simulink model "car_model"  (R2017a)
settings: Solver=ode8  StartTime=0.0  StopTime=tf  FixedStep=1e-3  RelTol=1e-3  AbsTol=1e-6
values from neighbouring files (symbols this model uses):
  L = sys.descrip.syms(end-2)    [load_consts.m]    (also in run_sim.m = sys.descrip.model_params(end-2))
  MAX_DELTA = deg2rad(MAX_DELTA)    [run_sim.m]
  w = sys.descrip.syms(end-3)    [load_consts.m]    (also in run_sim.m = sys.descrip.model_params(end-3))
  x0 = double(subs([qs0; ps0], symbs, vals))    [run_sim.m]
undefined symbols (not defined in the file or in its folder): sys
settings Model: Creator=brunolnetto  LastModifiedBy=brunolnetto
settings DataIOCC: SaveState=on  StateSaveName=xoutNew  OutputSaveName=youtNew

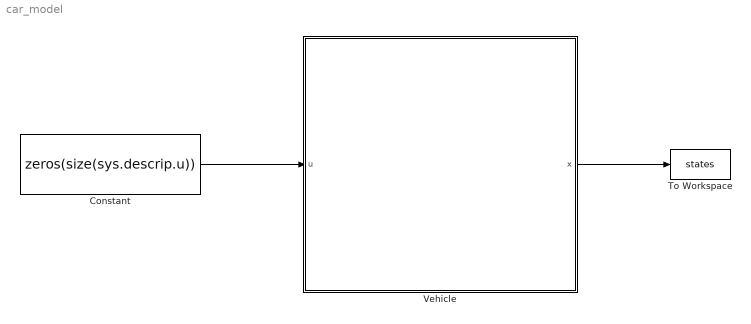
== system car_model ==
  Constant : Constant  Value=zeros(size(sys.descrip.u))
  To Workspace : ToWorkspace  VariableName=states  SaveFormat=Structure With Time  SampleTime=-1
  Vehicle : Subsystem
      mask Display: image('/home/brunolnetto/Pictures/auto_model.png');
  wires:
  Constant/1 -> Vehicle/1(u)
  Vehicle/1(x) -> To Workspace/1

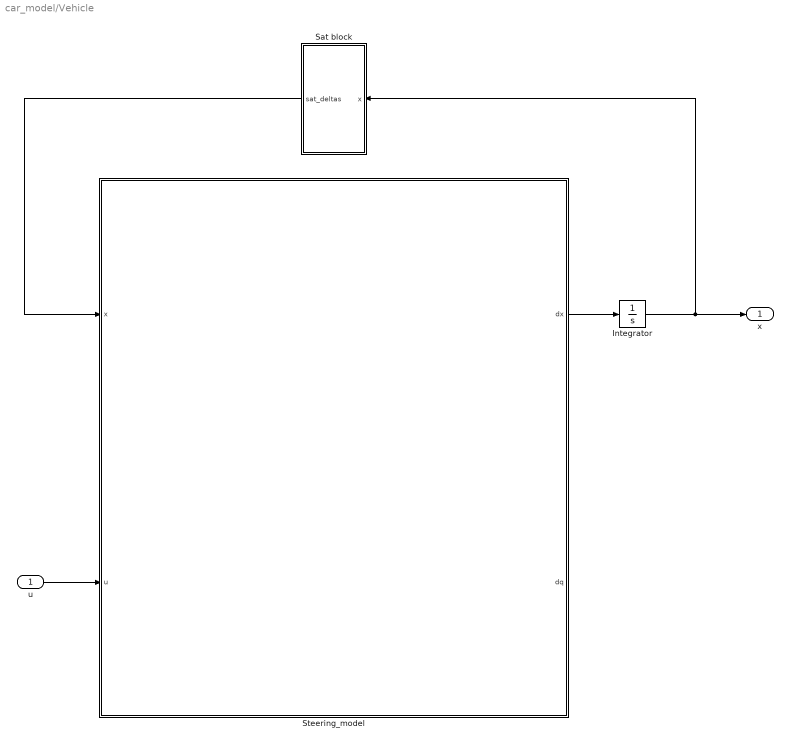
== system car_model/Vehicle ==
  u : Inport
  Integrator : Integrator  InitialCondition=x0
  Sat block : Subsystem
  Steering_model : Subsystem
      mask Display: image('/home/brunolnetto/Pictures/steer_schema.png');
  x : Outport
  wires:
  Steering_model/1(dx) -> Integrator/1
  u/1 -> Steering_model/2(u)
  Integrator/1 -> Sat block/1(x), x/1
  Sat block/1(sat_deltas) -> Steering_model/1(x)

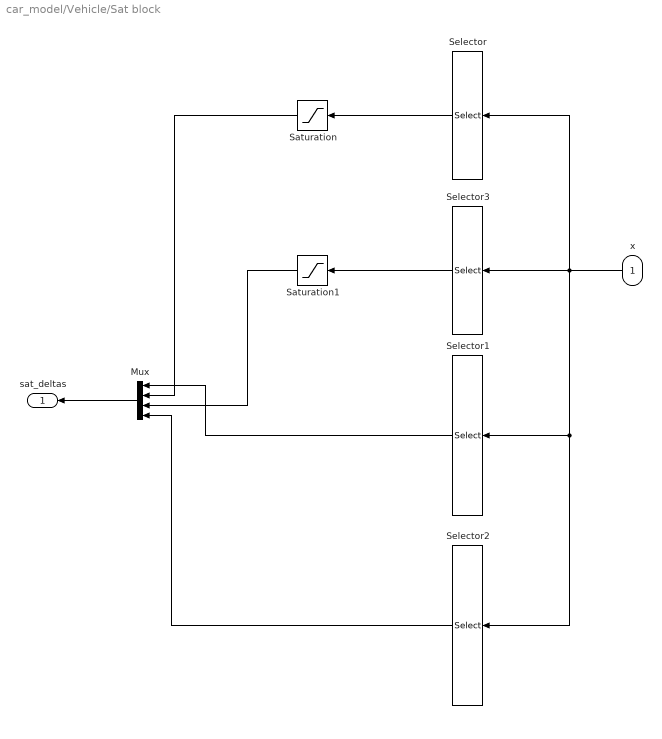
== system car_model/Vehicle/Sat block ==
  x : Inport
  Mux : Mux
  Saturation : Saturate  UpperLimit=MAX_DELTA  LowerLimit=atan(tan(-MAX_DELTA)/(1 - (w/L)*tan(-MAX_DELTA)))  LinearizeAsGain=off
  Saturation1 : Saturate  UpperLimit=atan(tan(MAX_DELTA)/(1 + (w/L)*tan(MAX_DELTA)))  LowerLimit=-MAX_DELTA  LinearizeAsGain=off
  Selector : Selector  InputPortWidth=length(x0)  IndexOptions=Index vector (dialog)  Indices=4  OutputSizes=1
  Selector1 : Selector  InputPortWidth=length(x0)  IndexOptions=Index vector (dialog)  Indices=[1 2. 3]  OutputSizes=1
  Selector2 : Selector  InputPortWidth=length(x0)  IndexOptions=Index vector (dialog)  Indices=6:length(x0)  OutputSizes=1
  Selector3 : Selector  InputPortWidth=length(x0)  IndexOptions=Index vector (dialog)  Indices=5  OutputSizes=1
  sat_deltas : Outport
  wires:
  Mux/1 -> sat_deltas/1
  x/1 -> Selector2/1, Selector1/1, Selector3/1, Selector/1
  Selector2/1 -> Mux/4
  Selector1/1 -> Mux/1
  Selector/1 -> Saturation/1
  Saturation/1 -> Mux/2
  Saturation1/1 -> Mux/3
  Selector3/1 -> Saturation1/1

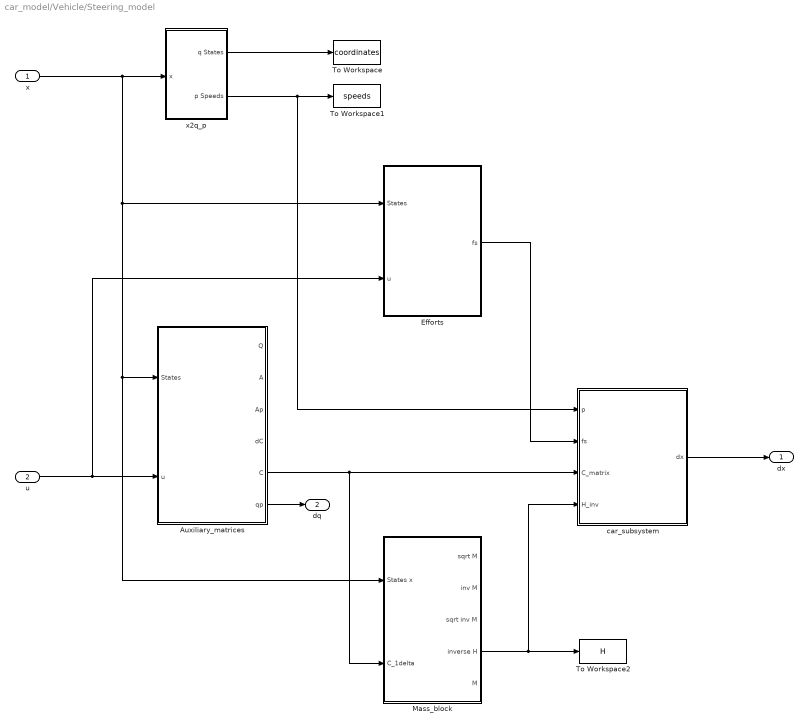
== system car_model/Vehicle/Steering_model ==
  x : Inport
  u : Inport  Port=2
  Auxiliary_matrices : Subsystem
  Efforts : Subsystem
  Mass_block : Subsystem
  To Workspace : ToWorkspace  VariableName=coordinates  SaveFormat=Structure With Time  SampleTime=-1
  To Workspace1 : ToWorkspace  VariableName=speeds  SaveFormat=Structure With Time  SampleTime=-1
  To Workspace2 : ToWorkspace  VariableName=H  SaveFormat=Structure With Time  SampleTime=-1
  car_subsystem : Subsystem
  x2q_p : Subsystem
  dx : Outport
  dq : Outport  Port=2
  wires:
  Auxiliary_matrices/5(C) -> Mass_block/2("C_1delta  "), car_subsystem/3(C_matrix)
  u/1 -> Efforts/2(u), Auxiliary_matrices/2(u)
  Mass_block/4(inverse H) -> To Workspace2/1, car_subsystem/4(H_inv)
  car_subsystem/1(dx) -> dx/1
  Efforts/1(fs) -> car_subsystem/2(fs)
  x2q_p/1(q States) -> To Workspace/1
  x2q_p/2(p Speeds) -> To Workspace1/1, car_subsystem/1(p)
  x/1 -> x2q_p/1(x), Mass_block/1(States x), Auxiliary_matrices/1(States), Efforts/1(States)
  Auxiliary_matrices/6(qp) -> dq/1

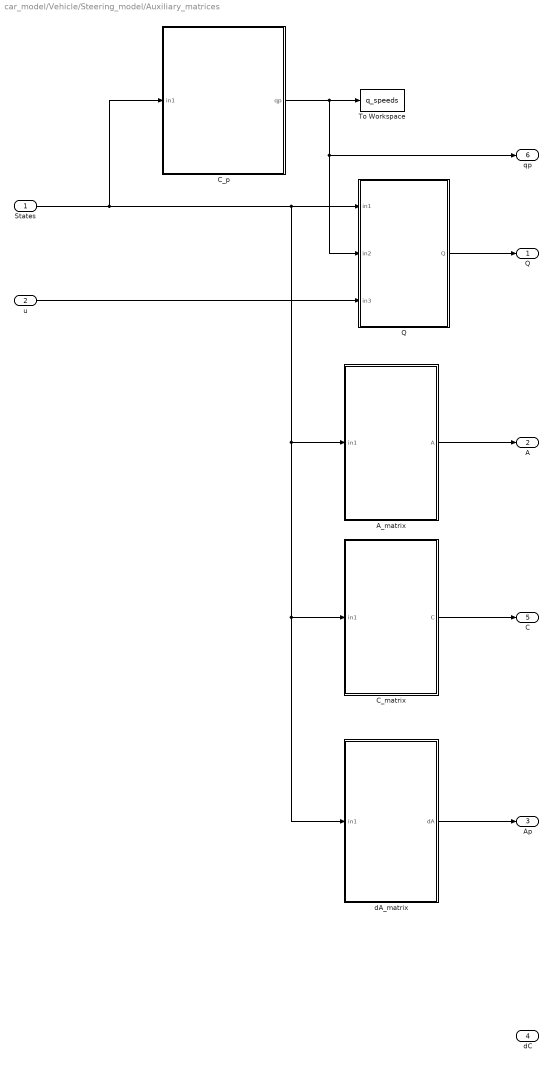
== system car_model/Vehicle/Steering_model/Auxiliary_matrices ==
  States : Inport
  u : Inport  Port=2
  A_matrix : MATLAB Function  TreatAsAtomicUnit=on
  C_matrix : MATLAB Function  TreatAsAtomicUnit=on
  C_p : MATLAB Function  TreatAsAtomicUnit=on
  Q : MATLAB Function  TreatAsAtomicUnit=on
  To Workspace : ToWorkspace  VariableName=q_speeds  SaveFormat=Structure With Time  SampleTime=-1
  dA_matrix : MATLAB Function  TreatAsAtomicUnit=on
  "Q " : Outport
  A : Outport  Port=2
  Ap : Outport  Port=3
  dC : Outport  Port=4
  C : Outport  Port=5
  qp : Outport  Port=6
  wires:
  C_matrix/1(C) -> C/1
  Q/1(Q) -> "Q "/1
  A_matrix/1(A) -> A/1
  dA_matrix/1(dA) -> Ap/1
  u/1 -> Q/3(in3)
  States/1 -> C_p/1(in1), dA_matrix/1(in1), C_matrix/1(in1), A_matrix/1(in1), Q/1(in1)
  C_p/1(qp) -> To Workspace/1, qp/1, Q/2(in2)

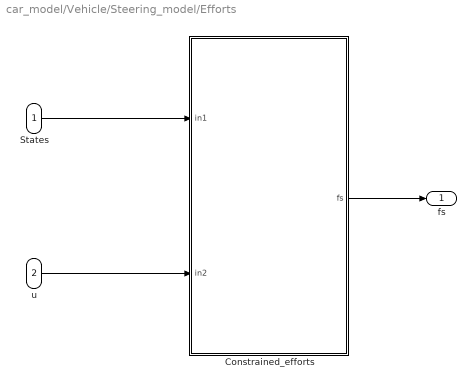
== system car_model/Vehicle/Steering_model/Efforts ==
  States : Inport
  u : Inport  Port=2
  Constrained_efforts : MATLAB Function  TreatAsAtomicUnit=on
  fs : Outport
  wires:
  States/1 -> Constrained_efforts/1(in1)
  u/1 -> Constrained_efforts/2(in2)
  Constrained_efforts/1(fs) -> fs/1

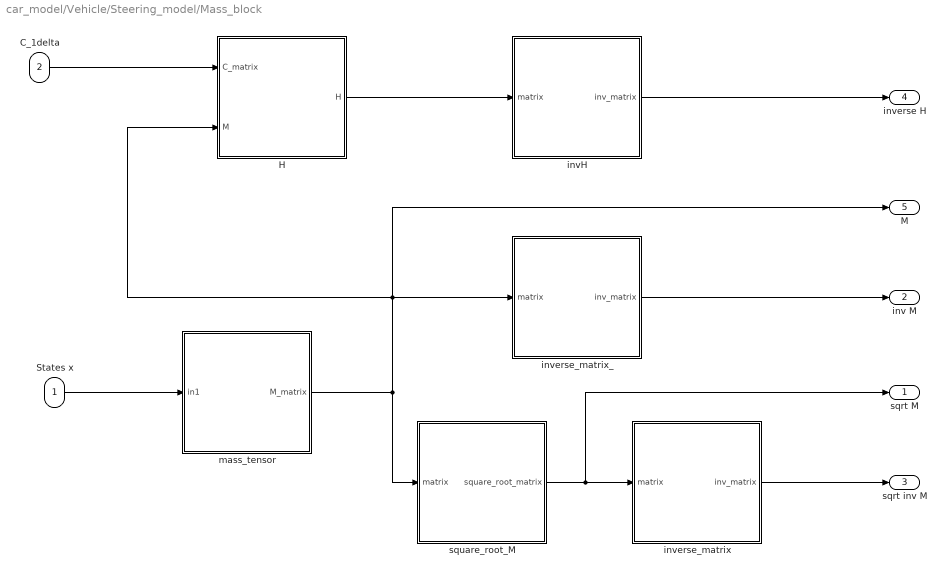
== system car_model/Vehicle/Steering_model/Mass_block ==
  States x : Inport
  "C_1delta  " : Inport  Port=2
  H : MATLAB Function  TreatAsAtomicUnit=on
  invH : MATLAB Function  TreatAsAtomicUnit=on
  inverse_matrix : MATLAB Function  TreatAsAtomicUnit=on
  inverse_matrix_ : MATLAB Function  TreatAsAtomicUnit=on
  mass_tensor : MATLAB Function  TreatAsAtomicUnit=on
  square_root_M : MATLAB Function  TreatAsAtomicUnit=on
  sqrt M : Outport
  inv M : Outport  Port=2
  sqrt inv M : Outport  Port=3
  inverse H : Outport  Port=4
  M : Outport  Port=5
  wires:
  States x/1 -> mass_tensor/1(in1)
  "C_1delta  "/1 -> H/1(C_matrix)
  inverse_matrix_/1(inv_matrix) -> inv M/1
  H/1(H) -> invH/1(matrix)
  invH/1(inv_matrix) -> inverse H/1
  inverse_matrix/1(inv_matrix) -> sqrt inv M/1
  mass_tensor/1(M_matrix) -> M/1, inverse_matrix_/1(matrix), H/2(M), square_root_M/1(matrix)
  square_root_M/1(square_root_matrix) -> sqrt M/1, inverse_matrix/1(matrix)

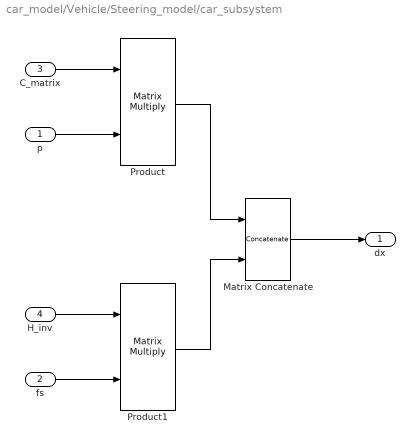
== system car_model/Vehicle/Steering_model/car_subsystem ==
  p : Inport
  fs : Inport  Port=2
  C_matrix : Inport  Port=3
  H_inv : Inport  Port=4
  Matrix Concatenate : Concatenate  ConcatenateDimension=2
  Product : Product  Multiplication=Matrix(*)
  Product1 : Product  Multiplication=Matrix(*)
  dx : Outport
  wires:
  Product/1 -> Matrix Concatenate/1
  p/1 -> Product/2
  C_matrix/1 -> Product/1
  Product1/1 -> Matrix Concatenate/2
  H_inv/1 -> Product1/1
  fs/1 -> Product1/2
  Matrix Concatenate/1 -> dx/1

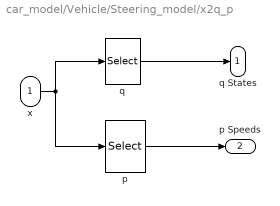
== system car_model/Vehicle/Steering_model/x2q_p ==
  x : Inport
  p : Selector  InputPortWidth=length(sys.kin.q) + length(sys.kin.p{end})  IndexOptions=Index vector (dialog)  Indices=length(sys.kin.q)+1:length(sys.kin.q) + length(sys.kin.p{end})  OutputSizes=1
  q : Selector  InputPortWidth=length(sys.kin.q) + length(sys.kin.p{end})  IndexOptions=Index vector (dialog)  Indices=1:length(sys.kin.q)  OutputSizes=1
  q States : Outport
  p Speeds : Outport  Port=2
  wires:
  x/1 -> p/1, q/1
  q/1 -> q States/1
  p/1 -> p Speeds/1

== matlab function car_model/Vehicle/Steering_model/Auxiliary_matrices/A_matrix ==
  data: in1 input; A output
function A = ConstraintMatrix(in1)

%    This function was generated by the Symbolic Math Toolbox version 7.2.

%    01-Dec-2020 16:45:13



delta_i = in1(4,:);

theta = in1(3,:);

t2 = tan(delta_i);

t3 = t2.*(3.0./2.0);

t4 = t3+9.0./2.0;

t5 = t2.^2;

t6 = t2.*(1.0./6.0);

t7 = t6+1.0;

t8 = 1.0./t7;

t9 = t2.*t8;

t10 = atan(t9);

t11 = t10.*2.0;

t12 = t11+theta;

t13 = 1.0./t4.^2;

t14 = t5.*t13.*(8.1e1./4.0);

t15 = t14+1.0;

t16 = cos(delta_i);

t17 = t16.*(9.0./2.0);

t18 = sin(delta_i);

t19 = t18.*(3.0./2.0);

t20 = t17+t19;

t21 = delta_i+theta;

t22 = sin(t21);

t23 = cos(t21);

A = reshape([0.0,cos(t12).*(-9.0./2.0)-cos(theta).*(9.0./2.0),0.0,0.0,0.0,t23,-t22,0.0,sin(t12).*(-9.0./2.0)-sin(theta).*(9.0./2.0),0.0,0.0,0.0,t22,t23,0.0,sin(t11).*(-8.1e1./8.0),0.0,0.0,0.0,-t17-t18.*(3.0./4.0),t16.*(-3.0./4.0)+t18.*(9.0./2.0),((t2.*(2.7e1./4.0))./t4-9.0./2.0).*(t5+1.0).*(-2.0./9.0),0.0,0.0,0.0,0.0,0.0,0.0,t4.*t15.*(-2.0./9.0),0.0,0.0,0.0,0.0,0.0,0.0,0.0,0.0,t20,0.0,t20,-3.442462000000001e-1,0.0,0.0,0.0,1.0./sqrt(t15).*(-9.0./2.0),0.0,0.0,0.0,0.0,0.0,0.0,0.0,-9.0./2.0,-9.0./2.0,0.0,0.0,0.0,t2.*5.163693000000001e-1+3.098215800000001,0.0,t4,0.0,0.0,0.0],[7,9]);

end

== matlab function car_model/Vehicle/Steering_model/Mass_block/mass_tensor ==
  data: in1 input; M_matrix output
function M_matrix = Mass_matrix(in1)

%    This function was generated by the Symbolic Math Toolbox version 7.2.

%    01-Dec-2020 16:45:20



phi_i = in1(6,:);

phi_l = in1(9,:);

phi_o = in1(7,:);

phi_r = in1(8,:);

theta = in1(3,:);

t2 = cos(theta);

t3 = sin(theta);

t4 = cos(phi_i);

t5 = cos(phi_l);

t6 = cos(phi_o);

t7 = cos(phi_r);

t8 = t4.^2;

t9 = sin(phi_i);

t10 = t6.^2;

t11 = sin(phi_o);

t12 = t8.*4.147690617505401e-1;

t13 = t9.^2;

t14 = t13.*2.073845308752701e-1;

t15 = t12+t14;

t16 = t10.*4.147690617505401e-1;

t17 = t11.^2;

t18 = t17.*2.073845308752701e-1;

t19 = t16+t18;

M_matrix = reshape([1.885e3,0.0,t2.*(-4.24125e3),0.0,0.0,0.0,0.0,0.0,0.0,0.0,1.885e3,t3.*(-4.24125e3),0.0,0.0,0.0,0.0,0.0,0.0,t2.*(-4.24125e3),t3.*(-4.24125e3),t8.*2.073845308752701e-1+t10.*2.073845308752701e-1+t5.^2.*2.073845308752701e-1+t7.^2.*2.073845308752701e-1+1.31830170381235e4,t15,t19,0.0,0.0,0.0,0.0,0.0,0.0,t15,t15,0.0,0.0,0.0,0.0,0.0,0.0,0.0,t19,0.0,t19,0.0,0.0,0.0,0.0,0.0,0.0,0.0,0.0,0.0,2.073845308752701e-1,0.0,0.0,0.0,0.0,0.0,0.0,0.0,0.0,0.0,2.073845308752701e-1,0.0,0.0,0.0,0.0,0.0,0.0,0.0,0.0,0.0,2.073845308752701e-1,0.0,0.0,0.0,0.0,0.0,0.0,0.0,0.0,0.0,2.073845308752701e-1],[9,9]);

end

== matlab function car_model/Vehicle/Steering_model/Auxiliary_matrices/C_matrix ==
  data: in1 input; C output
function C = KinematicMatrix(in1)

%    This function was generated by the Symbolic Math Toolbox version 7.2.

%    01-Dec-2020 16:45:15



delta_i = in1(4,:);

theta = in1(3,:);

t2 = sin(delta_i);

t3 = tan(delta_i);

t4 = delta_i+theta;

t5 = cos(delta_i);

t6 = sin(theta);

t7 = t3.^2;

t8 = t3.*(1.0./6.0);

t9 = t8+1.0;

t10 = 1.0./t9.^2;

t11 = t7.*t10;

t12 = t11+1.0;

t13 = 1.0./t12;

t14 = sin(t4);

t15 = cos(t4);

t16 = cos(theta);

t17 = t16.^2;

t18 = 1.0./t9;

t19 = t15.^2;

t20 = t14.^2;

t21 = t6.^2;

t22 = t5.^2;

t23 = t2.^2;

t24 = t5.*(9.0./2.0);

t25 = t2.*(3.0./2.0);

t26 = t24+t25;

t27 = 1.0./t26;

t28 = t5.*t6.*t13.*t14.*(8.1e1./2.0);

t29 = t2.*t13.*t14.*t16.*(8.1e1./2.0);

t30 = t2.*t6.*t13.*t14.*(2.7e1./4.0);

t31 = t5.*t13.*t15.*t16.*(8.1e1./2.0);

t32 = t5.*t6.*t13.*t15.*(2.7e1./4.0);

t33 = t2.*t13.*t15.*t16.*(2.7e1./4.0);

t34 = t3.*t13.*t17.*t18.*t19.*(8.1e1./4.0);

t35 = t3.*t13.*t17.*t18.*t20.*(8.1e1./4.0);

t36 = t3.*t13.*t18.*t19.*t21.*(8.1e1./4.0);

t37 = t3.*t13.*t18.*t20.*t21.*(8.1e1./4.0);

t38 = t3.*t5.*t13.*t15.*t16.*t18.*(2.7e1./4.0);

t39 = t3.*t5.*t13.*t14.*t16.*t18.*(8.1e1./2.0);

t40 = t3.*t5.*t6.*t13.*t14.*t18.*(2.7e1./4.0);

t41 = t2.*t3.*t13.*t14.*t16.*t18.*(2.7e1./4.0);

t44 = t2.*t6.*t13.*t15.*(8.1e1./2.0);

t45 = t5.*t13.*t14.*t16.*(2.7e1./4.0);

t46 = t3.*t5.*t6.*t13.*t15.*t18.*(8.1e1./2.0);

t47 = t2.*t3.*t13.*t15.*t16.*t18.*(8.1e1./2.0);

t48 = t2.*t3.*t6.*t13.*t15.*t18.*(2.7e1./4.0);

t49 = t2.*t3.*t6.*t13.*t14.*t18.*(8.1e1./2.0);

t42 = t28+t29+t30+t31+t32+t33+t34+t35+t36+t37+t38+t39+t40+t41-t44-t45-t46-t47-t48-t49;

t43 = 1.0./t42;

t50 = t3.*(3.0./2.0);

t51 = t50+9.0./2.0;

t52 = 1.0./t51;

t53 = 1.0./t51.^2;

C = reshape([0.0,0.0,0.0,(t50+t7.*t53.*(7.29e2./8.0)+t3.*t7.*t53.*(2.43e2./8.0)+9.0./2.0)./(t7.*(9.0./2.0)-t3.*t52.*(2.7e1./4.0)-t3.*t7.*t52.*(2.7e1./4.0)+9.0./2.0),1.0,0.0,0.0,0.0,0.0,t27.*t43.*(t14.*t22.*(-2.091295665e1)+t14.*t23.*4.182591330000001e1+t15.*t22.*1.254777399e2+t15.*t23.*6.970985550000001+t2.*t5.*t14.*1.1850675435e2-t2.*t6.*t13.*1.254777399e2+t2.*t5.*t15.*6.273886995000001e1+t5.*t6.*t13.*2.091295665e1-t3.*t14.*t22.*3.485492775000001+t3.*t14.*t23.*6.970985550000001+t3.*t15.*t22.*2.091295665e1+t3.*t15.*t23.*1.161830925+t2.*t3.*t5.*t14.*1.9751125725e1-t2.*t3.*t6.*t13.*4.182591330000001e1+t2.*t3.*t5.*t15.*1.0456478325e1+t3.*t5.*t6.*t13.*6.970985550000001-t2.*t3.*t13.*t16.*t18.*1.254777399e2+t3.*t5.*t13.*t16.*t18.*2.091295665e1-t2.*t7.*t13.*t16.*t18.*4.182591330000001e1+t5.*t7.*t13.*t16.*t18.*6.970985550000001+t3.*t13.*t15.*t17.*t18.*6.273886995000001e1+t3.*t13.*t15.*t18.*t21.*6.273886995000001e1+t7.*t13.*t15.*t17.*t18.*2.091295665e1+t7.*t13.*t15.*t18.*t21.*2.091295665e1).*(1.0./2.0),t27.*t43.*(t14.*t22.*(7.29e2./2.0)+t14.*t23.*(8.1e1./4.0)+t15.*t22.*(2.43e2./4.0)-t15.*t23.*(2.43e2./2.0)+t2.*t5.*t14.*(7.29e2./4.0)-t2.*t5.*t15.*3.4425e2+t2.*t13.*t16.*(7.29e2./2.0)-t5.*t13.*t16.*(2.43e2./4.0)+t3.*t14.*t22.*(2.43e2./4.0)+t3.*t14.*t23.*(2.7e1./8.0)+t3.*t15.*t22.*(8.1e1./8.0)-t3.*t15.*t23.*(8.1e1./4.0)+t2.*t3.*t5.*t14.*(2.43e2./8.0)-t2.*t3.*t5.*t15.*(4.59e2./8.0)+t2.*t3.*t13.*t16.*(2.43e2./2.0)-t3.*t5.*t13.*t16.*(8.1e1./4.0)-t2.*t3.*t6.*t13.*t18.*(7.29e2./2.0)+t3.*t5.*t6.*t13.*t18.*(2.43e2./4.0)-t2.*t6.*t7.*t13.*t18.*(2.43e2./2.0)+t5.*t6.*t7.*t13.*t18.*(8.1e1./4.0)+t3.*t13.*t14.*t17.*t18.*(7.29e2./4.0)+t3.*t13.*t14.*t18.*t21.*(7.29e2./4.0)+t7.*t13.*t14.*t17.*t18.*(2.43e2./4.0)+t7.*t13.*t14.*t18.*t21.*(2.43e2./4.0)).*1.721231e-1,t27.*t43.*(t2.*t19.*(2.7e1./2.0)+t2.*t20.*(2.7e1./2.0)+t5.*t19.*(8.1e1./2.0)+t5.*t20.*(8.1e1./2.0)+t2.*t3.*t19.*(9.0./4.0)+t2.*t3.*t20.*(9.0./4.0)+t3.*t5.*t19.*(2.7e1./4.0)+t3.*t5.*t20.*(2.7e1./4.0)-t6.*t13.*t14.*(8.1e1./2.0)-t13.*t15.*t16.*(8.1e1./2.0)-t3.*t6.*t13.*t14.*(2.7e1./2.0)-t3.*t13.*t15.*t16.*(2.7e1./2.0)+t3.*t6.*t13.*t15.*t18.*(8.1e1./2.0)+t6.*t7.*t13.*t15.*t18.*(2.7e1./2.0)-t3.*t13.*t14.*t16.*t18.*(8.1e1./2.0)-t7.*t13.*t14.*t16.*t18.*(2.7e1./2.0)).*3.442462000000001e-1,0.0,0.0,t27.*t51,t51.*sqrt(t7.*t53.*(8.1e1./4.0)+1.0).*(2.0./9.0),t3.*(1.0./3.0)+1.0,1.0],[9,2]);

end

== matlab function car_model/Vehicle/Steering_model/Auxiliary_matrices/Q ==
  data: in1 input; in2 input; in3 input; Q output
function Q = EffortVector(in1,in2,in3)

%    This function was generated by the Symbolic Math Toolbox version 7.2.

%    01-Dec-2020 16:45:13



deltap_i = in2(4,:);

deltap_o = in2(5,:);

f_phi_i = in3(1,:);

f_phi_l = in3(4,:);

f_phi_o = in3(2,:);

f_phi_r = in3(3,:);

phi_i = in1(6,:);

phi_l = in1(9,:);

phi_o = in1(7,:);

phi_r = in1(8,:);

phip_i = in2(6,:);

phip_l = in2(9,:);

phip_o = in2(7,:);

phip_r = in2(8,:);

thetap = in2(3,:);

theta = in1(3,:);

t2 = thetap.^2;

t3 = phi_i.*2.0;

t4 = sin(t3);

t5 = phi_o.*2.0;

t6 = sin(t5);

t7 = deltap_i+thetap;

t8 = deltap_o+thetap;

t9 = phi_r.*2.0;

t10 = sin(t9);

t11 = phi_l.*2.0;

t12 = sin(t11);

Q = [t2.*sin(theta).*(-4.24125e3);t2.*cos(theta).*4.24125e3;deltap_i.*phip_i.*t4.*2.073845308752701e-1+deltap_o.*phip_o.*t6.*2.073845308752701e-1+phip_i.*t4.*thetap.*2.073845308752701e-1+phip_o.*t6.*thetap.*2.073845308752701e-1+phip_l.*t12.*thetap.*2.073845308752701e-1+phip_r.*t10.*thetap.*2.073845308752701e-1;phip_i.*(deltap_i.*t4.*2.073845308752701e-1+t4.*thetap.*2.073845308752701e-1);phip_o.*(deltap_o.*t6.*2.073845308752701e-1+t6.*thetap.*2.073845308752701e-1);f_phi_i-t4.*t7.^2.*1.03692265437635e-1;f_phi_o-t6.*t8.^2.*1.03692265437635e-1;f_phi_r-t2.*t10.*1.03692265437635e-1;f_phi_l-t2.*t12.*1.03692265437635e-1];

end

== matlab function car_model/Vehicle/Steering_model/Auxiliary_matrices/dA_matrix ==
  data: in1 input; dA output
function dA = dConstraintMatrix(in1)

%    This function was generated by the Symbolic Math Toolbox version 7.2.

%    01-Dec-2020 16:45:19



delta_i = in1(4,:);

p1 = in1(10,:);

p2 = in1(11,:);

theta = in1(3,:);

t2 = tan(delta_i);

t3 = t2.*(3.0./2.0);

t4 = t3+9.0./2.0;

t5 = t2.^2;

t6 = t5+1.0;

t7 = 1.0./t4;

t8 = t2.*t7.*(2.7e1./4.0);

t9 = 1.0./t4.^2;

t10 = t5.*(9.0./2.0);

t11 = t2.*t5.*t7.*(2.7e1./4.0);

t12 = t8-t10+t11-9.0./2.0;

t13 = 1.0./t12;

t14 = t5.*t9.*(7.29e2./8.0);

t15 = t2.*t5.*t9.*(2.43e2./8.0);

t16 = t3+t14+t15+9.0./2.0;

t19 = delta_i+theta;

t17 = cos(t19);

t18 = cos(delta_i);

t20 = sin(t19);

t21 = t17.^2;

t22 = sin(delta_i);

t23 = t20.^2;

t24 = t2.*(1.0./6.0);

t25 = t24+1.0;

t26 = sin(theta);

t27 = 1.0./t25.^2;

t28 = t5.*t27;

t29 = t28+1.0;

t30 = 1.0./t29;

t31 = cos(theta);

t32 = 1.0./t25;

t33 = t31.^2;

t34 = t26.^2;

t35 = t2.*t32;

t36 = atan(t35);

t37 = t36.*2.0;

t38 = t37+theta;

t39 = sin(t38);

t40 = t18.*(9.0./2.0);

t41 = t22.*(3.0./2.0);

t42 = t40+t41;

t43 = 1.0./t42;

t44 = t18.*t21.*(8.1e1./2.0);

t45 = t18.*t23.*(8.1e1./2.0);

t46 = t21.*t22.*(2.7e1./2.0);

t47 = t22.*t23.*(2.7e1./2.0);

t48 = t2.*t18.*t23.*(2.7e1./4.0);

t49 = t2.*t21.*t22.*(9.0./4.0);

t50 = t2.*t22.*t23.*(9.0./4.0);

t51 = t2.*t18.*t21.*(2.7e1./4.0);

t52 = t2.*t17.*t26.*t30.*t32.*(8.1e1./2.0);

t53 = t5.*t17.*t26.*t30.*t32.*(2.7e1./2.0);

t83 = t17.*t30.*t31.*(8.1e1./2.0);

t84 = t20.*t26.*t30.*(8.1e1./2.0);

t85 = t2.*t20.*t26.*t30.*(2.7e1./2.0);

t86 = t2.*t17.*t30.*t31.*(2.7e1./2.0);

t87 = t2.*t20.*t30.*t31.*t32.*(8.1e1./2.0);

t88 = t5.*t20.*t30.*t31.*t32.*(2.7e1./2.0);

t54 = t44+t45+t46+t47+t48+t49+t50+t51+t52+t53-t83-t84-t85-t86-t87-t88;

t55 = t18.*t20.*t26.*t30.*(8.1e1./2.0);

t56 = t20.*t22.*t30.*t31.*(8.1e1./2.0);

t57 = t20.*t22.*t26.*t30.*(2.7e1./4.0);

t58 = t17.*t18.*t30.*t31.*(8.1e1./2.0);

t59 = t17.*t18.*t26.*t30.*(2.7e1./4.0);

t60 = t17.*t22.*t30.*t31.*(2.7e1./4.0);

t61 = t2.*t21.*t30.*t32.*t33.*(8.1e1./4.0);

t62 = t2.*t23.*t30.*t32.*t33.*(8.1e1./4.0);

t63 = t2.*t21.*t30.*t32.*t34.*(8.1e1./4.0);

t64 = t2.*t23.*t30.*t32.*t34.*(8.1e1./4.0);

t65 = t2.*t17.*t18.*t30.*t31.*t32.*(2.7e1./4.0);

t66 = t2.*t18.*t20.*t30.*t31.*t32.*(8.1e1./2.0);

t67 = t2.*t18.*t20.*t26.*t30.*t32.*(2.7e1./4.0);

t68 = t2.*t20.*t22.*t30.*t31.*t32.*(2.7e1./4.0);

t89 = t17.*t22.*t26.*t30.*(8.1e1./2.0);

t90 = t18.*t20.*t30.*t31.*(2.7e1./4.0);

t91 = t2.*t17.*t18.*t26.*t30.*t32.*(8.1e1./2.0);

t92 = t2.*t17.*t22.*t30.*t31.*t32.*(8.1e1./2.0);

t93 = t2.*t17.*t22.*t26.*t30.*t32.*(2.7e1./4.0);

t94 = t2.*t20.*t22.*t26.*t30.*t32.*(8.1e1./2.0);

t69 = t55+t56+t57+t58+t59+t60+t61+t62+t63+t64+t65+t66+t67+t68-t89-t90-t91-t92-t93-t94;

t70 = 1.0./t69;

t71 = cos(t38);

t72 = t6.*t32;

t74 = t2.*t6.*t27.*(1.0./6.0);

t73 = t72-t74;

t75 = 1.0./t4.^3;

t76 = t2.*t6.*t9.*(8.1e1./2.0);

t77 = t5.*t9.*(8.1e1./4.0);

t78 = t77+1.0;

t79 = t76-t5.*t6.*t75.*(2.43e2./4.0);

t80 = t18.*(3.0./2.0);

t81 = t22.*(9.0./2.0);

t82 = t80-t81;

t95 = p2.*t17.*t43.*t54.*t70.*3.442462000000001e-1;

t96 = p1.*t13.*t16.*t20;

t97 = t96-p2.*t20.*t43.*t54.*t70.*3.442462000000001e-1;

dA = reshape([0.0,p2.*t43.*t54.*t70.*(t26+t39).*1.5491079-p1.*t13.*t16.*t30.*t39.*t73.*9.0,0.0,0.0,0.0,t97,-t95+p1.*t13.*t16.*t17,0.0,p2.*t43.*t54.*t70.*(t31+t71).*(-1.5491079)+p1.*t13.*t16.*t30.*t71.*t73.*9.0,0.0,0.0,0.0,t95-p1.*t13.*t16.*t17,t97,0.0,p1.*t13.*t16.*t30.*t73.*cos(t37).*(8.1e1./4.0),0.0,0.0,0.0,p1.*t13.*t16.*(t18.*(3.0./4.0)-t81),-p1.*t13.*t16.*(t22.*(3.0./4.0)+t40),p1.*t13.*t16.*(t6.*(t6.*t7.*(2.7e1./4.0)-t2.*t6.*t9.*(8.1e1./8.0)).*(2.0./9.0)+t2.*t6.*(t8-9.0./2.0).*(4.0./9.0)),0.0,0.0,0.0,0.0,0.0,0.0,p1.*t13.*t16.*(t4.*t79.*(2.0./9.0)+t6.*t78.*(1.0./3.0)),0.0,0.0,0.0,0.0,0.0,0.0,0.0,0.0,-p1.*t13.*t16.*t82,0.0,-p1.*t13.*t16.*t82,0.0,0.0,0.0,0.0,p1.*t13.*t16.*1.0./t78.^(3.0./2.0).*t79.*(-9.0./4.0),0.0,0.0,0.0,0.0,0.0,0.0,0.0,0.0,0.0,0.0,0.0,0.0,p1.*t6.*t13.*t16.*(-5.163693000000001e-1),0.0,p1.*t6.*t13.*t16.*(-3.0./2.0),0.0,0.0,0.0],[7,9]);

end

== matlab function car_model/Vehicle/Steering_model/Efforts/Constrained_efforts ==
  data: in1 input; in2 input; fs output
function fs = ConstrainedEffort(in1,in2)

%    This function was generated by the Symbolic Math Toolbox version 7.2.

%    01-Dec-2020 16:45:27



delta_i = in1(4,:);

delta_o = in1(5,:);

f_phi_i = in2(1,:);

f_phi_l = in2(4,:);

f_phi_o = in2(2,:);

f_phi_r = in2(3,:);

p1 = in1(10,:);

p2 = in1(11,:);

phi_i = in1(6,:);

phi_l = in1(9,:);

phi_o = in1(7,:);

phi_r = in1(8,:);

theta = in1(3,:);

t2 = phi_o.*2.0;

t3 = sin(t2);

t6 = delta_i+theta;

t4 = cos(t6);

t5 = cos(delta_i);

t7 = sin(t6);

t8 = t4.^2;

t9 = sin(delta_i);

t10 = t7.^2;

t11 = tan(delta_i);

t12 = t11.^2;

t13 = t11.*(1.0./6.0);

t14 = t13+1.0;

t15 = 1.0./t14.^2;

t16 = t12.*t15;

t17 = t16+1.0;

t18 = 1.0./t17;

t19 = sin(theta);

t20 = cos(theta);

t21 = 1.0./t14;

t22 = t20.^2;

t23 = t19.^2;

t24 = t11.*(3.0./2.0);

t25 = t24+9.0./2.0;

t26 = 1.0./t25;

t27 = 1.0./t25.^2;

t28 = phi_i.*2.0;

t29 = sin(t28);

t30 = t5.*(9.0./2.0);

t31 = t9.*(3.0./2.0);

t32 = t30+t31;

t33 = 1.0./t32;

t34 = t5.*t8.*(8.1e1./2.0);

t35 = t5.*t10.*(8.1e1./2.0);

t36 = t8.*t9.*(2.7e1./2.0);

t37 = t9.*t10.*(2.7e1./2.0);

t38 = t5.*t10.*t11.*(2.7e1./4.0);

t39 = t8.*t9.*t11.*(9.0./4.0);

t40 = t9.*t10.*t11.*(9.0./4.0);

t41 = t5.*t8.*t11.*(2.7e1./4.0);

t42 = t4.*t11.*t18.*t19.*t21.*(8.1e1./2.0);

t43 = t4.*t12.*t18.*t19.*t21.*(2.7e1./2.0);

t70 = t4.*t18.*t20.*(8.1e1./2.0);

t71 = t7.*t18.*t19.*(8.1e1./2.0);

t72 = t7.*t11.*t18.*t19.*(2.7e1./2.0);

t73 = t4.*t11.*t18.*t20.*(2.7e1./2.0);

t74 = t7.*t11.*t18.*t20.*t21.*(8.1e1./2.0);

t75 = t7.*t12.*t18.*t20.*t21.*(2.7e1./2.0);

t44 = t34+t35+t36+t37+t38+t39+t40+t41+t42+t43-t70-t71-t72-t73-t74-t75;

t45 = t5.*t7.*t18.*t19.*(8.1e1./2.0);

t46 = t7.*t9.*t18.*t20.*(8.1e1./2.0);

t47 = t7.*t9.*t18.*t19.*(2.7e1./4.0);

t48 = t4.*t5.*t18.*t20.*(8.1e1./2.0);

t49 = t4.*t5.*t18.*t19.*(2.7e1./4.0);

t50 = t4.*t9.*t18.*t20.*(2.7e1./4.0);

t51 = t8.*t11.*t18.*t21.*t22.*(8.1e1./4.0);

t52 = t10.*t11.*t18.*t21.*t22.*(8.1e1./4.0);

t53 = t8.*t11.*t18.*t21.*t23.*(8.1e1./4.0);

t54 = t10.*t11.*t18.*t21.*t23.*(8.1e1./4.0);

t55 = t4.*t5.*t11.*t18.*t20.*t21.*(2.7e1./4.0);

t56 = t5.*t7.*t11.*t18.*t20.*t21.*(8.1e1./2.0);

t57 = t5.*t7.*t11.*t18.*t19.*t21.*(2.7e1./4.0);

t58 = t7.*t9.*t11.*t18.*t20.*t21.*(2.7e1./4.0);

t76 = t4.*t9.*t18.*t19.*(8.1e1./2.0);

t77 = t5.*t7.*t18.*t20.*(2.7e1./4.0);

t78 = t4.*t5.*t11.*t18.*t19.*t21.*(8.1e1./2.0);

t79 = t4.*t9.*t11.*t18.*t20.*t21.*(8.1e1./2.0);

t80 = t4.*t9.*t11.*t18.*t19.*t21.*(2.7e1./4.0);

t81 = t7.*t9.*t11.*t18.*t19.*t21.*(8.1e1./2.0);

t59 = t45+t46+t47+t48+t49+t50+t51+t52+t53+t54+t55+t56+t57+t58-t76-t77-t78-t79-t80-t81;

t60 = 1.0./t59;

t61 = t12.*(9.0./2.0);

t68 = t11.*t26.*(2.7e1./4.0);

t69 = t11.*t12.*t26.*(2.7e1./4.0);

t62 = t61-t68-t69+9.0./2.0;

t63 = 1.0./t62;

t64 = t12.*t27.*(7.29e2./8.0);

t65 = t11.*t12.*t27.*(2.43e2./8.0);

t66 = t24+t64+t65+9.0./2.0;

t67 = 1.0./t5;

t83 = p2.*t33.*t44.*t60.*3.442462000000001e-1;

t82 = t83+p1.*t63.*t66;

t84 = p1+t83;

t85 = t12.*t27.*(8.1e1./4.0);

t86 = t85+1.0;

t87 = sqrt(t86);

t88 = p2.^2;

t89 = phi_l.*2.0;

t90 = sin(t89);

t91 = 1.0./t32.^2;

t92 = phi_r.*2.0;

t93 = sin(t92);

t94 = t44.^2;

t95 = 1.0./t59.^2;

t96 = t5.^2;

t97 = t9.^2;

t98 = 1.0./t32.^3;

t99 = 1.0./t59.^3;

fs = [p2.*t25.*t87.*(p1.*t3.*2.073845308752701e-1+p2.*t3.*t33.*t44.*t60.*7.13913366925944e-2).*(2.0./9.0)+p2.*t25.*t33.*t63.*t66.*(p1.*t29.*t63.*t66.*2.073845308752701e-1+p2.*t29.*t33.*t44.*t60.*7.13913366925944e-2);f_phi_l+f_phi_i.*t67+f_phi_r.*(t9.*t67.*(1.0./3.0)+1.0)-t25.*t29.*t33.*t82.^2.*1.03692265437635e-1-t3.*t25.*t84.^2.*t87.*2.304272565280778e-2+(f_phi_o.*t32.*t67.*(2.0./9.0))./cos(delta_o)+t33.*t44.*t60.*(p1.*p2.*t3.*t25.*t87.*4.608545130561557e-2+t33.*t44.*t60.*t88.*t90.*7.13913366925944e-2+t25.*t29.*t44.*t60.*t88.*t91.*7.13913366925944e-2+t25.*t33.*t44.*t60.*t88.*t93.*1.58647414872432e-2+p1.*p2.*t25.*t29.*t33.*t63.*t66.*2.073845308752701e-1+t3.*t25.*t33.*t44.*t60.*t87.*t88.*1.58647414872432e-2).*3.442462000000001e-1-t88.*t90.*t91.*t94.*t95.*1.22880981846731e-2-t25.*t88.*t91.*t93.*t94.*t95.*2.730688485482911e-3+t20.*t88.*t94.*t98.*t99.*(t4.*t96.*(2.43e2./4.0)-t4.*t97.*(2.43e2./2.0)+t7.*t96.*(7.29e2./2.0)+t7.*t97.*(8.1e1./4.0)-t4.*t5.*t9.*3.4425e2+t5.*t7.*t9.*(7.29e2./4.0)-t5.*t18.*t20.*(2.43e2./4.0)+t9.*t18.*t20.*(7.29e2./2.0)+t4.*t11.*t96.*(8.1e1./8.0)-t4.*t11.*t97.*(8.1e1./4.0)+t7.*t11.*t96.*(2.43e2./4.0)+t7.*t11.*t97.*(2.7e1./8.0)-t4.*t5.*t9.*t11.*(4.59e2./8.0)+t5.*t7.*t9.*t11.*(2.43e2./8.0)-t5.*t11.*t18.*t20.*(8.1e1./4.0)+t9.*t11.*t18.*t20.*(2.43e2./2.0)+t5.*t11.*t18.*t19.*t21.*(2.43e2./4.0)+t5.*t12.*t18.*t19.*t21.*(8.1e1./4.0)-t9.*t11.*t18.*t19.*t21.*(7.29e2./2.0)+t7.*t11.*t18.*t21.*t22.*(7.29e2./4.0)-t9.*t12.*t18.*t19.*t21.*(2.43e2./2.0)+t7.*t11.*t18.*t21.*t23.*(7.29e2./4.0)+t7.*t12.*t18.*t21.*t22.*(2.43e2./4.0)+t7.*t12.*t18.*t21.*t23.*(2.43e2./4.0)).*8.651100192784744e1-t19.*t88.*t94.*t98.*t99.*(t4.*t96.*1.254777399e2+t4.*t97.*6.970985550000001-t7.*t96.*2.091295665e1+t7.*t97.*4.182591330000001e1+t4.*t5.*t9.*6.273886995000001e1+t5.*t7.*t9.*1.1850675435e2+t5.*t18.*t19.*2.091295665e1-t9.*t18.*t19.*1.254777399e2+t4.*t11.*t96.*2.091295665e1+t4.*t11.*t97.*1.161830925-t7.*t11.*t96.*3.485492775000001+t7.*t11.*t97.*6.970985550000001+t4.*t5.*t9.*t11.*1.0456478325e1+t5.*t7.*t9.*t11.*1.9751125725e1+t5.*t11.*t18.*t19.*6.970985550000001-t9.*t11.*t18.*t19.*4.182591330000001e1+t5.*t11.*t18.*t20.*t21.*2.091295665e1+t4.*t11.*t18.*t21.*t22.*6.273886995000001e1+t5.*t12.*t18.*t20.*t21.*6.970985550000001+t4.*t11.*t18.*t21.*t23.*6.273886995000001e1+t4.*t12.*t18.*t21.*t22.*2.091295665e1+t4.*t12.*t18.*t21.*t23.*2.091295665e1-t9.*t11.*t18.*t20.*t21.*1.254777399e2-t9.*t12.*t18.*t20.*t21.*4.182591330000001e1).*2.513056118784969e2];

end

== matlab function car_model/Vehicle/Steering_model/Mass_block/H ==
  data: C_matrix input; H output; M input
function H = ConstrinedMassMatrix(C_matrix, M)
% MASSMATRIX
%    This function was generated by the Symbolic Math Toolbox version 7.2.
%    16-Oct-2020 11:55:07

    H = C_matrix'*M*C_matrix;
end

== matlab function car_model/Vehicle/Steering_model/Mass_block/invH ==
  data: matrix input; inv_matrix output
function inv_matrix = matrix_inverse(matrix)
% MASSMATRIX
%    This function was generated by the Symbolic Math Toolbox version 7.2.
%    16-Oct-2020 11:55:07

    inv_matrix = inv(matrix);
end

== matlab function car_model/Vehicle/Steering_model/Mass_block/inverse_matrix_ ==
  data: matrix input; inv_matrix output
function inv_matrix = matrix_inverse(matrix)
% MASSMATRIX
%    This function was generated by the Symbolic Math Toolbox version 7.2.
%    16-Oct-2020 11:55:07

    inv_matrix = inv(matrix);
end

== matlab function car_model/Vehicle/Steering_model/Mass_block/square_root_M ==
  data: matrix input; square_root_matrix output
function square_root_matrix = matrix_square_root(matrix)
% MASSMATRIX
%    This function was generated by the Symbolic Math Toolbox version 7.2.
%    16-Oct-2020 11:55:07

    square_root_matrix = real(sqrtm(matrix));
end

== matlab function car_model/Vehicle/Steering_model/Mass_block/inverse_matrix ==
  data: matrix input; inv_matrix output
function inv_matrix = matrix_inverse(matrix)
% MASSMATRIX
%    This function was generated by the Symbolic Math Toolbox version 7.2.
%    16-Oct-2020 11:55:07

    inv_matrix = inv(matrix);
end

== matlab function car_model/Vehicle/Steering_model/Auxiliary_matrices/C_p ==
  data: in1 input; qp output
function qp = KinematicVector(in1)

%    This function was generated by the Symbolic Math Toolbox version 7.2.

%    01-Dec-2020 16:45:12



delta_i = in1(4,:);

p1 = in1(10,:);

p2 = in1(11,:);

theta = in1(3,:);

t2 = sin(delta_i);

t3 = tan(delta_i);

t4 = delta_i+theta;

t5 = cos(delta_i);

t6 = sin(theta);

t7 = t3.^2;

t8 = t3.*(1.0./6.0);

t9 = t8+1.0;

t10 = 1.0./t9.^2;

t11 = t7.*t10;

t12 = t11+1.0;

t13 = 1.0./t12;

t14 = sin(t4);

t15 = cos(t4);

t16 = cos(theta);

t17 = t16.^2;

t18 = 1.0./t9;

t19 = t15.^2;

t20 = t14.^2;

t21 = t6.^2;

t22 = t5.^2;

t23 = t2.^2;

t24 = t5.*(9.0./2.0);

t25 = t2.*(3.0./2.0);

t26 = t24+t25;

t27 = 1.0./t26;

t28 = t5.*t6.*t13.*t14.*(8.1e1./2.0);

t29 = t2.*t13.*t14.*t16.*(8.1e1./2.0);

t30 = t2.*t6.*t13.*t14.*(2.7e1./4.0);

t31 = t5.*t13.*t15.*t16.*(8.1e1./2.0);

t32 = t5.*t6.*t13.*t15.*(2.7e1./4.0);

t33 = t2.*t13.*t15.*t16.*(2.7e1./4.0);

t34 = t3.*t13.*t17.*t18.*t19.*(8.1e1./4.0);

t35 = t3.*t13.*t17.*t18.*t20.*(8.1e1./4.0);

t36 = t3.*t13.*t18.*t19.*t21.*(8.1e1./4.0);

t37 = t3.*t13.*t18.*t20.*t21.*(8.1e1./4.0);

t38 = t3.*t5.*t13.*t15.*t16.*t18.*(2.7e1./4.0);

t39 = t3.*t5.*t13.*t14.*t16.*t18.*(8.1e1./2.0);

t40 = t3.*t5.*t6.*t13.*t14.*t18.*(2.7e1./4.0);

t41 = t2.*t3.*t13.*t14.*t16.*t18.*(2.7e1./4.0);

t44 = t2.*t6.*t13.*t15.*(8.1e1./2.0);

t45 = t5.*t13.*t14.*t16.*(2.7e1./4.0);

t46 = t3.*t5.*t6.*t13.*t15.*t18.*(8.1e1./2.0);

t47 = t2.*t3.*t13.*t15.*t16.*t18.*(8.1e1./2.0);

t48 = t2.*t3.*t6.*t13.*t15.*t18.*(2.7e1./4.0);

t49 = t2.*t3.*t6.*t13.*t14.*t18.*(8.1e1./2.0);

t42 = t28+t29+t30+t31+t32+t33+t34+t35+t36+t37+t38+t39+t40+t41-t44-t45-t46-t47-t48-t49;

t43 = 1.0./t42;

t50 = t3.*(3.0./2.0);

t51 = t50+9.0./2.0;

t52 = 1.0./t51;

t53 = 1.0./t51.^2;

qp = [p2.*t27.*t43.*(t14.*t22.*(-2.091295665e1)+t14.*t23.*4.182591330000001e1+t15.*t22.*1.254777399e2+t15.*t23.*6.970985550000001+t2.*t5.*t14.*1.1850675435e2-t2.*t6.*t13.*1.254777399e2+t2.*t5.*t15.*6.273886995000001e1+t5.*t6.*t13.*2.091295665e1-t3.*t14.*t22.*3.485492775000001+t3.*t14.*t23.*6.970985550000001+t3.*t15.*t22.*2.091295665e1+t3.*t15.*t23.*1.161830925+t2.*t3.*t5.*t14.*1.9751125725e1-t2.*t3.*t6.*t13.*4.182591330000001e1+t2.*t3.*t5.*t15.*1.0456478325e1+t3.*t5.*t6.*t13.*6.970985550000001-t2.*t3.*t13.*t16.*t18.*1.254777399e2+t3.*t5.*t13.*t16.*t18.*2.091295665e1-t2.*t7.*t13.*t16.*t18.*4.182591330000001e1+t5.*t7.*t13.*t16.*t18.*6.970985550000001+t3.*t13.*t15.*t17.*t18.*6.273886995000001e1+t3.*t13.*t15.*t18.*t21.*6.273886995000001e1+t7.*t13.*t15.*t17.*t18.*2.091295665e1+t7.*t13.*t15.*t18.*t21.*2.091295665e1).*(1.0./2.0);p2.*t27.*t43.*(t14.*t22.*(7.29e2./2.0)+t14.*t23.*(8.1e1./4.0)+t15.*t22.*(2.43e2./4.0)-t15.*t23.*(2.43e2./2.0)+t2.*t5.*t14.*(7.29e2./4.0)-t2.*t5.*t15.*3.4425e2+t2.*t13.*t16.*(7.29e2./2.0)-t5.*t13.*t16.*(2.43e2./4.0)+t3.*t14.*t22.*(2.43e2./4.0)+t3.*t14.*t23.*(2.7e1./8.0)+t3.*t15.*t22.*(8.1e1./8.0)-t3.*t15.*t23.*(8.1e1./4.0)+t2.*t3.*t5.*t14.*(2.43e2./8.0)-t2.*t3.*t5.*t15.*(4.59e2./8.0)+t2.*t3.*t13.*t16.*(2.43e2./2.0)-t3.*t5.*t13.*t16.*(8.1e1./4.0)-t2.*t3.*t6.*t13.*t18.*(7.29e2./2.0)+t3.*t5.*t6.*t13.*t18.*(2.43e2./4.0)-t2.*t6.*t7.*t13.*t18.*(2.43e2./2.0)+t5.*t6.*t7.*t13.*t18.*(8.1e1./4.0)+t3.*t13.*t14.*t17.*t18.*(7.29e2./4.0)+t3.*t13.*t14.*t18.*t21.*(7.29e2./4.0)+t7.*t13.*t14.*t17.*t18.*(2.43e2./4.0)+t7.*t13.*t14.*t18.*t21.*(2.43e2./4.0)).*1.721231e-1;p2.*t27.*t43.*(t2.*t19.*(2.7e1./2.0)+t2.*t20.*(2.7e1./2.0)+t5.*t19.*(8.1e1./2.0)+t5.*t20.*(8.1e1./2.0)+t2.*t3.*t19.*(9.0./4.0)+t2.*t3.*t20.*(9.0./4.0)+t3.*t5.*t19.*(2.7e1./4.0)+t3.*t5.*t20.*(2.7e1./4.0)-t6.*t13.*t14.*(8.1e1./2.0)-t13.*t15.*t16.*(8.1e1./2.0)-t3.*t6.*t13.*t14.*(2.7e1./2.0)-t3.*t13.*t15.*t16.*(2.7e1./2.0)+t3.*t6.*t13.*t15.*t18.*(8.1e1./2.0)+t6.*t7.*t13.*t15.*t18.*(2.7e1./2.0)-t3.*t13.*t14.*t16.*t18.*(8.1e1./2.0)-t7.*t13.*t14.*t16.*t18.*(2.7e1./2.0)).*3.442462000000001e-1;(p1.*(t50+t7.*t53.*(7.29e2./8.0)+t3.*t7.*t53.*(2.43e2./8.0)+9.0./2.0))./(t7.*(9.0./2.0)-t3.*t52.*(2.7e1./4.0)-t3.*t7.*t52.*(2.7e1./4.0)+9.0./2.0);p1;p2.*t27.*t51;p2.*t51.*sqrt(t7.*t53.*(8.1e1./4.0)+1.0).*(2.0./9.0);p2.*t51.*(2.0./9.0);p2];

end
